simulink library "VehicleDynamics"  (R2024a)
settings: Solver=VariableStepAuto  StartTime=0.0  StopTime=10.0  RelTol=1e-3
values from neighbouring files (symbols this model uses):
  GearRatio = 0.275    [VehicleDynamics.sldd]
  WheelRadius = 8.0    [VehicleDynamics.sldd]
undefined symbols (not defined in the file or in its folder): raptor_xcp_function
libraries: Raptor_lib x3
settings Model: Creator=serga  LastModifiedBy=serga

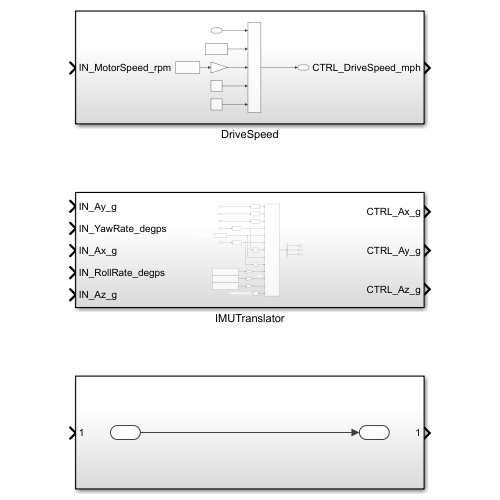
[thumbnail: Simulink's stored preview of the top-level diagram]
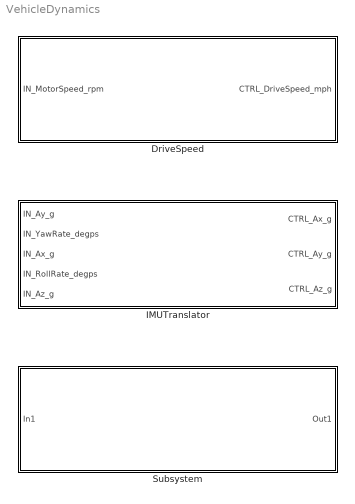
== system VehicleDynamics ==
  DriveSpeed : Subsystem
  IMUTranslator : Subsystem
  Subsystem : Subsystem

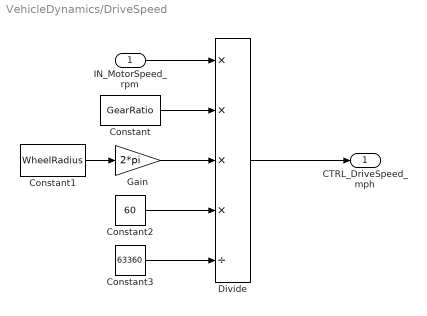
== system VehicleDynamics/DriveSpeed ==
  IN_MotorSpeed_rpm : Inport
  Constant : Constant  Value=GearRatio
  Constant1 : Constant  Value=WheelRadius
  Constant2 : Constant  Value=60
  Constant3 : Constant  Value=63360
  Divide : Product  Inputs=****/  RndMeth=Zero  SaturateOnIntegerOverflow=on
  Gain : Gain  Gain=2*pi
  CTRL_DriveSpeed_mph : Outport
  wires:
  Divide/1 -> CTRL_DriveSpeed_mph/1
  Constant3/1 -> Divide/5
  Constant2/1 -> Divide/4
  Gain/1 -> Divide/3
  Constant1/1 -> Gain/1
  Constant/1 -> Divide/2
  IN_MotorSpeed_rpm/1 -> Divide/1

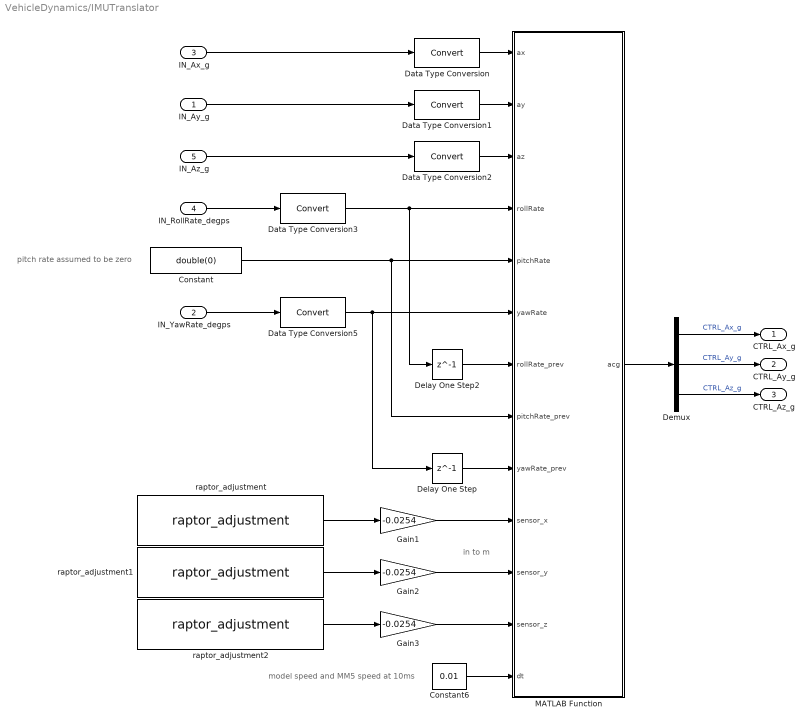
== system VehicleDynamics/IMUTranslator ==
  note: model speed and MM5 speed at 10ms
  note: pitch rate assumed to be zero
  note: in to m
  IN_Ay_g : Inport
  IN_YawRate_degps : Inport  Port=2
  IN_Ax_g : Inport  Port=3
  IN_RollRate_degps : Inport  Port=4
  IN_Az_g : Inport  Port=5
  Constant : Constant  Value=double(0)
  Constant6 : Constant  Value=0.01
  Data Type Conversion{,1..3,5} (5 alike) : DataTypeConversion  SaturateOnIntegerOverflow=off  RndMeth=Floor
  Delay One Step : Delay  DelayLength=1
  Delay One Step2 : Delay  DelayLength=1
  Demux : Demux  Outputs=3
  Gain1 : Gain  Gain=-0.0254
  Gain2 : Gain  Gain=-0.0254
  Gain3 : Gain  Gain=-0.0254
  MATLAB Function : MATLAB Function  TreatAsAtomicUnit=on
  raptor_adjustment : Raptor_lib/Data Storage/raptor_adjustment  paramName='CTRL_MM5XOffset_in'  nameSource=Parameter  initValue=-40.55  dataType=double  storage=Calibration  calDispType=Number  calEnum={'False', 'True'}  calGain=1.0  calOffset=0.0  calMax=inf  calMin=-inf  calFormat='-1'  calUnit=''  calHelp=''  calAccess=1  calFunction=raptor_xcp_function(gcb)  calDispHeaders=off  calColHeaders={'Col1' 'Col2' 'Col3'}  calRowHeaders={'Row1' 'Row2' 'Row3'}
      settings: SourceProductName=Raptor
  raptor_adjustment1 : Raptor_lib/Data Storage/raptor_adjustment  paramName='CTRL_MM5YOffset_in'  nameSource=Parameter  initValue=0  dataType=double  storage=Calibration  calDispType=Number  calEnum={'False', 'True'}  calGain=1.0  calOffset=0.0  calMax=inf  calMin=-inf  calFormat='-1'  calUnit=''  calHelp=''  calAccess=1  calFunction=raptor_xcp_function(gcb)  calDispHeaders=off  calColHeaders={'Col1' 'Col2' 'Col3'}  calRowHeaders={'Row1' 'Row2' 'Row3'}
      settings: SourceProductName=Raptor
  raptor_adjustment2 : Raptor_lib/Data Storage/raptor_adjustment  paramName='CTRL_MM5ZOffset_in'  nameSource=Parameter  initValue=-12  dataType=double  storage=Calibration  calDispType=Number  calEnum={'False', 'True'}  calGain=1.0  calOffset=0.0  calMax=inf  calMin=-inf  calFormat='-1'  calUnit=''  calHelp=''  calAccess=1  calFunction=raptor_xcp_function(gcb)  calDispHeaders=off  calColHeaders={'Col1' 'Col2' 'Col3'}  calRowHeaders={'Row1' 'Row2' 'Row3'}
      settings: SourceProductName=Raptor
  CTRL_Ax_g : Outport
  CTRL_Ay_g : Outport  Port=2
  CTRL_Az_g : Outport  Port=3
  wires:
  Data Type Conversion5/1 -> Delay One Step/1, MATLAB Function/6(yawRate)
  Data Type Conversion3/1 -> Delay One Step2/1, MATLAB Function/4(rollRate)
  IN_YawRate_degps/1 -> Data Type Conversion5/1
  Constant/1 -> MATLAB Function/8(pitchRate_prev), MATLAB Function/5(pitchRate)
  IN_RollRate_degps/1 -> Data Type Conversion3/1
  Data Type Conversion2/1 -> MATLAB Function/3(az)
  Data Type Conversion1/1 -> MATLAB Function/2(ay)
  Data Type Conversion/1 -> MATLAB Function/1(ax)
  Demux/3 -> CTRL_Az_g/1  "CTRL_Az_g"
  Demux/2 -> CTRL_Ay_g/1  "CTRL_Ay_g"
  Demux/1 -> CTRL_Ax_g/1  "CTRL_Ax_g"
  MATLAB Function/1(acg) -> Demux/1
  IN_Ax_g/1 -> Data Type Conversion/1
  IN_Az_g/1 -> Data Type Conversion2/1
  Gain3/1 -> MATLAB Function/12(sensor_z)
  Gain2/1 -> MATLAB Function/11(sensor_y)
  Gain1/1 -> MATLAB Function/10(sensor_x)
  IN_Ay_g/1 -> Data Type Conversion1/1
  Delay One Step2/1 -> MATLAB Function/7(rollRate_prev)
  Delay One Step/1 -> MATLAB Function/9(yawRate_prev)
  Constant6/1 -> MATLAB Function/13(dt)
  raptor_adjustment2/1 -> Gain3/1
  raptor_adjustment1/1 -> Gain2/1
  raptor_adjustment/1 -> Gain1/1

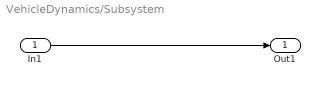
== system VehicleDynamics/Subsystem ==
  In1 : Inport
  Out1 : Outport
  wires:
  In1/1 -> Out1/1

== matlab function VehicleDynamics/IMUTranslator/MATLAB Function ==
  data: ax input; ay input; az input; rollRate input; acg output; pitchRate input; yawRate input; rollRate_prev input; pitchRate_prev input; yawRate_prev input; sensor_x input; sensor_y input; sensor_z input; dt input
function acg = fcn(ax, ay, az, rollRate, pitchRate, yawRate, rollRate_prev,...
    pitchRate_prev, yawRate_prev, sensor_x, sensor_y, sensor_z, dt)

% gravity vector (gravity already in az)
% g = [0; 0; -9.80665];

% sensor to cg
r = [sensor_x; sensor_y; sensor_z];

% accelerometer data from sensor (g to m/s^2)
accel_meas = [ax; ay; az] * 9.80665;

% gyroscope data from sensor (deg/s to rad/s)
omega = [rollRate; pitchRate; yawRate] * 0.01745;

% previous gyroscope data from sensor (deg/s to rad/s)
omega_prev = [rollRate_prev; pitchRate_prev; yawRate_prev] * 0.01745;

% angular acceleration (m/s^2)
alpha = (omega - omega_prev)/dt;

% rotational contributions (m/s^2)
centripetal = cross(omega, cross(omega, r));

tangential = cross(alpha, r);

 % cg acceleration in chassis frame (m/s^2)
% acgm = accel_meas + g - tangential - centripetal;
acgm = accel_meas - tangential - centripetal;

% m/s^2 to g
acg = acgm * 0.10197;
